simulink model "VentilatorModel_v3_Lyb"  (R2017b)
settings: Solver=ode23tb  StartTime=0.0  StopTime=30  FixedStep=0.001  MaxStep=0.005  RelTol=1e-6  EnableMultiTasking=on
undefined symbols (not defined in the file or in its folder): InputData
libraries: Simple_pneu_library x2
settings Model: Creator=ferossi  LastModifiedBy=upattacini
settings SolverCC: MaxConsecutiveMinStep=100
settings DataIOCC: SaveFormat=Array
settings OptimizationCC: LifeSpan=inf
settings DebuggingCC: SolverPrmCheckMsg=warning  SFUnexpectedBacktrackingDiag=warning  SFNoUnconditionalDefaultTransitionDiag=warning  SFExecutionAtInitializationDiag=none
settings HardwareCC: ProdBitPerPointer=32  ProdBitPerSizeT=32  ProdBitPerPtrDiffT=32  ProdLargestAtomicFloat=None  ProdIntDivRoundTo=Undefined  ProdEndianess=Unspecified  ProdWordSize=32  ProdHWDeviceType=32-bit Generic
settings ModelReferenceCC: PropagateSignalLabelsOutOfModel=off
settings CodeAppCC: StateflowObjectComments=on
settings GRTTargetCC: TargetLangStandard=C89/C90 (ANSI)
settings ConfigComp: CovMetricSettings=dw  CovHtmlReporting=on  CovSaveCumulativeToWorkspaceVar=on  CovSaveSingleToWorkspaceVar=on  CovExternalEMLEnable=off  CovSFcnEnable=off

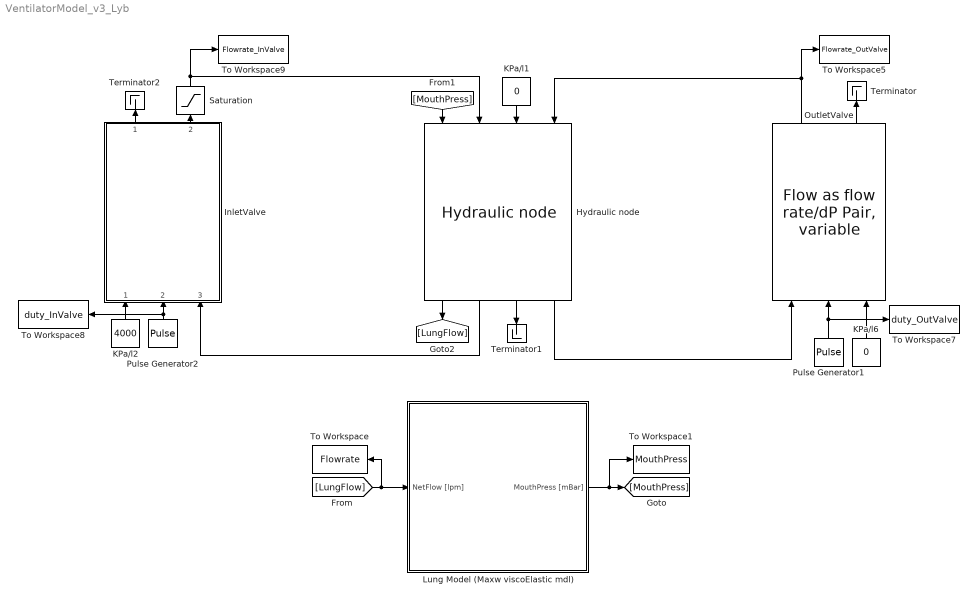
== system VentilatorModel_v3_Lyb ==
  Hydraulic node : Simple_pneu_library/Hydraulic node  SystemSampleTime=-1  Latency=0  AutoFrameSizeCalculation=off
  InletValve : Subsystem  mask{dp=InputData.InValve.BrkPress, flow=InputData.InValve.Data, posizione=InputData.InValve.BrkDuty}
      mask prompts: dp "Reference Pressure Drop [mbar]"; flow "Flow Rate [L/min]"; posizione "Duty [%]"
  KPa/l1 : Constant  Value=0
  KPa/l2 : Constant  Value=4000
  KPa/l6 : Constant  Value=0
  Lung Model (Maxw viscoElastic mdl) : Subsystem  mask{Stiff1=100, Stiff2=2.6, Damp=0.9, R0=0.47, Kv=-0.45, Kf=0.01}
      mask prompts: Stiff1 "Stiffness in series with damp"; Stiff2 "Stiffness in parallel"; Damp "Damping"; R0 "Laminar flow resistance"; Kv "Volum resistance coeff"; Kf "Flow resistance coeff"
      mask Display: image('../assets/lung.png');
  OutletValve : Simple_pneu_library/Flow as flow rate//dP Pair, variable  dp=InputData.OutValve.BrkPress  flow=InputData.OutValve.Data
  Pulse Generator1 : DiscretePulseGenerator  PulseType=Time based  Amplitude=InputData.OutValve.DutyMax  Period=InputData.InValve.Period  PulseWidth=InputData.OutValve.PulseWidth  PhaseDelay=2.1
  Pulse Generator2 : DiscretePulseGenerator  PulseType=Time based  Amplitude=InputData.InValve.DutyMax  Period=InputData.InValve.Period  PulseWidth=InputData.InValve.PulseWidth
  Saturation : Saturate  UpperLimit=1000  LowerLimit=0
  Terminator : Terminator
  Terminator1 : Terminator
  Terminator2 : Terminator
  To Workspace : ToWorkspace  VariableName=Flowrate  SampleTime=-1
  To Workspace1 : ToWorkspace  VariableName=MouthPress  SampleTime=-1
  To Workspace5 : ToWorkspace  VariableName=Flowrate_OutValve  SampleTime=-1
  To Workspace7 : ToWorkspace  VariableName=duty_OutValve  SampleTime=-1
  To Workspace8 : ToWorkspace  VariableName=duty_InValve  SampleTime=-1
  To Workspace9 : ToWorkspace  VariableName=Flowrate_InValve  SampleTime=-1
  wires:
  [LungFlow] -> To Workspace/1, Lung Model (Maxw viscoElastic mdl)/1(NetFlow [lpm])
  Lung Model (Maxw viscoElastic mdl)/1(MouthPress [mBar]) -> [MouthPress], To Workspace1/1
  KPa/l6/1 -> OutletValve/3
  Pulse Generator1/1 -> To Workspace7/1, OutletValve/2
  OutletValve/2 -> Terminator/1
  KPa/l1/1 -> Hydraulic node/3
  Hydraulic node/3 -> Terminator1/1
  OutletValve/1 -> Hydraulic node/4, To Workspace5/1
  Hydraulic node/4 -> OutletValve/1
  [MouthPress] -> Hydraulic node/1
  Hydraulic node/1 -> [LungFlow]
  InletValve/1("Flow rate port 1 ") -> Terminator2/1
  InletValve/2("Flow rate port 2 ") -> Saturation/1
  KPa/l2/1 -> InletValve/1("Pressure port 1 ")
  Pulse Generator2/1 -> To Workspace8/1, InletValve/2(Valve position)
  Hydraulic node/2 -> InletValve/3(Pressure port 2)
  Saturation/1 -> To Workspace9/1, Hydraulic node/2

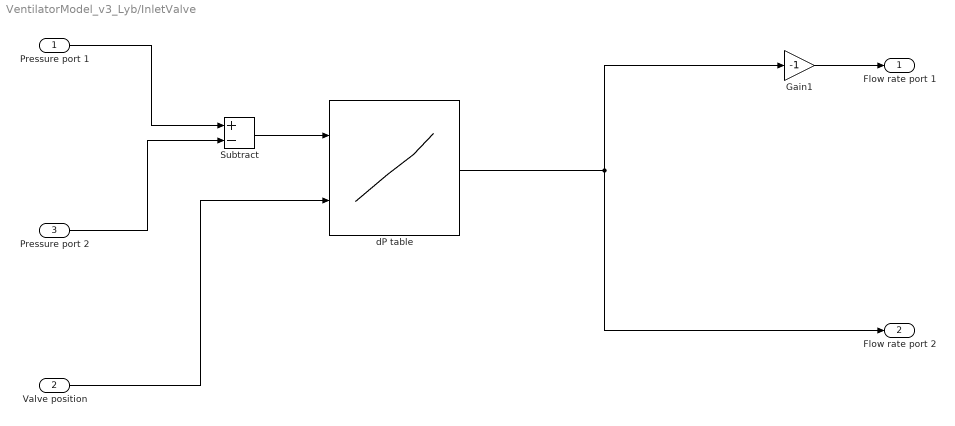
== system VentilatorModel_v3_Lyb/InletValve ==
  "Pressure port 1 " : Inport
  Valve position : Inport  Port=2
  Pressure port 2 : Inport  Port=3
  Gain1 : Gain  Gain=-1
  Subtract : Sum  Inputs=+-
  dP table : Lookup_n-D  BreakpointsForDimension1=dp  BreakpointsForDimension2=posizione  BeginIndexSearchUsingPreviousIndexResult=on  Table=flow  InternalRulePriority=Speed  RndMeth=Simplest  InputSameDT=on
  "Flow rate port 1 " : Outport  VectorParamsAs1DForOutWhenUnconnected=off
  "Flow rate port 2 " : Outport  Port=2  VectorParamsAs1DForOutWhenUnconnected=off
  wires:
  dP table/1 -> Gain1/1, "Flow rate port 2 "/1
  Valve position/1 -> dP table/2
  Pressure port 2/1 -> Subtract/2
  Gain1/1 -> "Flow rate port 1 "/1
  Subtract/1 -> dP table/1
  "Pressure port 1 "/1 -> Subtract/1

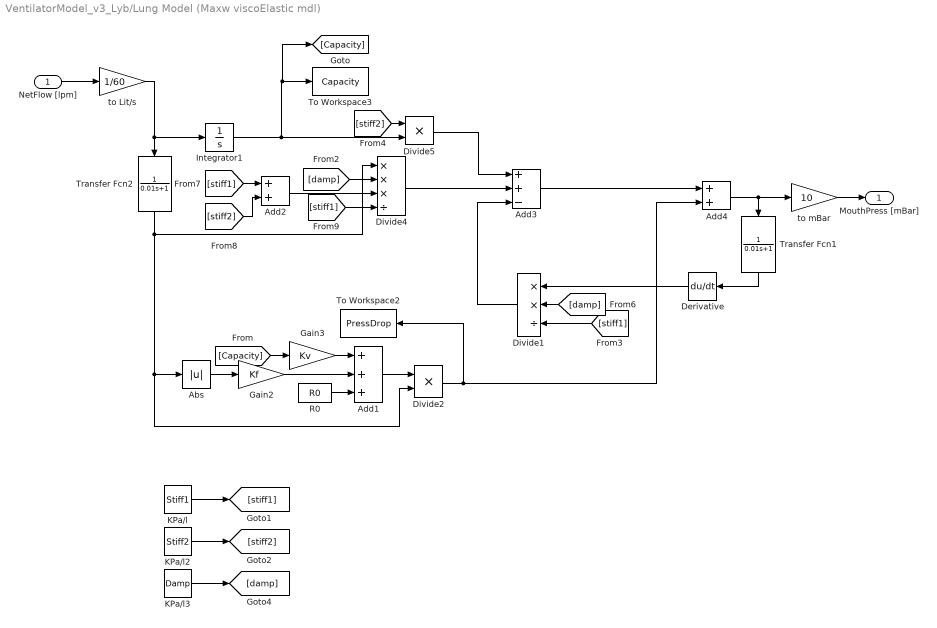
== system VentilatorModel_v3_Lyb/Lung Model (Maxw viscoElastic mdl) ==
  NetFlow [lpm] : Inport
  Abs : Abs
  Add1 : Sum  Inputs=+++
  Add2 : Sum
  Add3 : Sum  Inputs=++-
  Add4 : Sum
  Derivative : Derivative
  Divide1 : Product  Inputs=**/
  Divide2 : Product  Inputs=**
  Divide4 : Product  Inputs=***/
  Divide5 : Product  Inputs=**
  Gain2 : Gain  Gain=Kf
  Gain3 : Gain  Gain=Kv
  Integrator1 : Integrator
  KPa/l : Constant  Value=Stiff1
  KPa/l2 : Constant  Value=Stiff2
  KPa/l3 : Constant  Value=Damp
  R0 : Constant  Value=R0
  To Workspace2 : ToWorkspace  VariableName=PressDrop  SampleTime=-1
  To Workspace3 : ToWorkspace  VariableName=Capacity  SampleTime=-1
  Transfer Fcn1 : TransferFcn  Denominator=[0.01 1]
  Transfer Fcn2 : TransferFcn  Denominator=[0.01 1]
  to Lit/s : Gain  Gain=1/60
  to mBar : Gain  Gain=10
  MouthPress [mBar] : Outport  VectorParamsAs1DForOutWhenUnconnected=off
  wires:
  NetFlow [lpm]/1 -> to Lit/s/1
  Add3/1 -> Add4/1
  Add4/1 -> Transfer Fcn1/1, to mBar/1
  KPa/l3/1 -> [damp]
  R0/1 -> Add1/3
  KPa/l/1 -> [stiff1]
  Abs/1 -> Gain2/1
  Gain3/1 -> Add1/1
  Add1/1 -> Divide2/1
  [stiff1] -> Add2/1
  Gain2/1 -> Add1/2
  [damp] -> Divide1/2
  Divide5/1 -> Add3/1
  [stiff1] -> Divide1/3
  to Lit/s/1 -> Transfer Fcn2/1, Integrator1/1
  [stiff2] -> Add2/2
  Divide2/1 -> Add4/2, To Workspace2/1
  [stiff1] -> Divide4/4
  Divide1/1 -> Add3/3
  Divide4/1 -> Add3/2
  Integrator1/1 -> Divide5/2, [Capacity], To Workspace3/1
  [damp] -> Divide4/2
  Derivative/1 -> Divide1/1
  [stiff2] -> Divide5/1
  KPa/l2/1 -> [stiff2]
  [Capacity] -> Gain3/1
  Add2/1 -> Divide4/3
  to mBar/1 -> MouthPress [mBar]/1
  Transfer Fcn1/1 -> Derivative/1
  Transfer Fcn2/1 -> Abs/1, Divide2/2, Divide4/1
